simulink model "square"  (R2015a)
settings: Solver=ode45  StartTime=0.0  StopTime=0.1  MaxStep=1e-6  RelTol=1e-3
libraries: powerlib x8
settings Model: Creator=KP SINGH  LastModifiedBy=KP SINGH

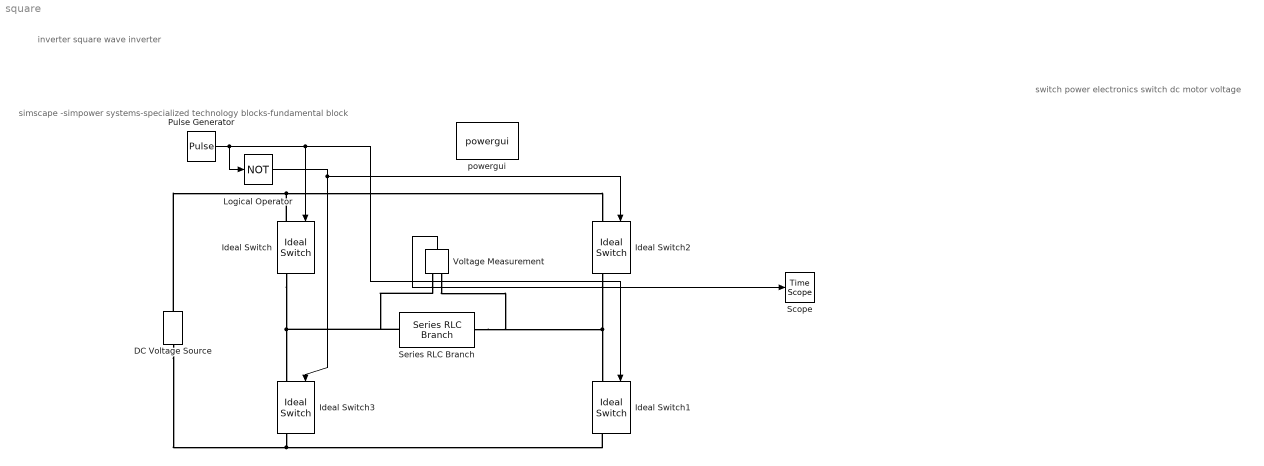
== system square ==
  note: simscape -simpower systems-specialized technology blocks-fundamental block
  note: switch power electronics
      | switch dc motor voltage
  note: inverter
      | square wave inverter
  DC Voltage Source : powerlib/Electrical Sources/DC Voltage Source  Amplitude=100  Measurements=None
  Ideal Switch{,1..3} (4 alike) : powerlib/Power Electronics/Ideal Switch  Ron=0.001  Lon=0  IC=0  Rs=1e5  Cs=inf  Measurements=on
  Logical Operator : Logic  Operator=NOT  IconShape=distinctive  AllPortsSameDT=off  OutDataTypeStr=boolean
  Pulse Generator : DiscretePulseGenerator  PulseType=Time based  Period=0.02  PulseWidth=50
  Scope : TimeScope
  Series RLC Branch : powerlib/Elements/Series RLC Branch  LConnTagsString=__new0  RConnTagsString=__new0  BranchType=R  Resistance=100  Inductance=1e-3  SetiL0=off  InitialCurrent=0  Capacitance=1e-6  Setx0=off  InitialVoltage=0  Measurements=None
  Voltage Measurement : powerlib/Measurements/Voltage Measurement  PhasorSimulation=off  OutputType=Complex  PSBequivalent=0
  powergui : powerlib/powergui  Priority=1  SimulationMode=Continuous  SolverType=Tustin/Backward Euler (TBE)  SampleTime=50e-6  frequency=60  SPID=off  DisableSnubberDevices=off  DisableRonSwitches=off  DisableVfSwitches=off  SwTol=0  DisplayEquations=off  Interpol=off  methode=off  Ts=100  FunctionMessages=off  echomessages=off  HookPort=off  EnableUseOfTLC=off  x0status=blocks  frequencyindice=0  Pbase=100e6  ErrMax=1e-4  Iterations=50  UnitsV=kV  UnitsW=MW  buscounter=0  RestoreLinks=warning  ResistiveCurrentMeasurement=off  Frange=[0:2:500]  Ylog=off  Xlog=on  ShowGrid=off  save=off  variable=ZData  structure=0  ZoomFFT=off  StartTime=0.0  cycles=1  DisplayStyle=1  fundamental=60  FreqAxis=off  MaxFrequency=1000  frequencyindicesteady=1  RmsSteady=1  display=off
  wires:
  Voltage Measurement/1 -> Scope/1
  Pulse Generator/1 -> Logical Operator/1, Ideal Switch1/1, Ideal Switch/1
  Logical Operator/1 -> Ideal Switch2/1, Ideal Switch3/1
  connections:
  Ideal Switch/LConn1 -- DC Voltage Source/RConn1 -- Ideal Switch2/LConn1
  Ideal Switch/RConn1 -- Voltage Measurement/LConn1 -- Series RLC Branch/LConn1 -- Ideal Switch3/LConn1
  Ideal Switch2/RConn1 -- Voltage Measurement/LConn2 -- Series RLC Branch/RConn1 -- Ideal Switch1/LConn1
  Ideal Switch3/RConn1 -- Ideal Switch1/RConn1 -- DC Voltage Source/LConn1
